simulink model "FootVelocityCalculator"  (R2016b)
settings: Solver=VariableStepAuto  StartTime=0.0  StopTime=10.0  RelTol=1e-3
settings Model: DataDictionary=DataDictionary.sldd  Creator=Taeke  LastModifiedBy=Nathan

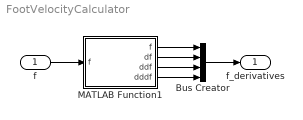
== system FootVelocityCalculator ==
  f : Inport  PortDimensions=numberSamplePoints
  Bus Creator : BusCreator  Inputs='f','df','ddf','dddf'  OutDataTypeStr=Bus: hip
  MATLAB Function1 : MATLAB Function  TreatAsAtomicUnit=on
  f_derivatives : Outport  OutDataTypeStr=Bus: hip
  wires:
  MATLAB Function1/1(f) -> Bus Creator/1
  MATLAB Function1/3(ddf) -> Bus Creator/3
  MATLAB Function1/2(df) -> Bus Creator/2
  MATLAB Function1/4(dddf) -> Bus Creator/4
  f/1 -> MATLAB Function1/1("f ")
  Bus Creator/1 -> f_derivatives/1

== matlab function FootVelocityCalculator/MATLAB Function1 ==
  data: f input; f output; df output; ddf output; dddf output

function [f, df, ddf, dddf] = fcn(f)
t = 0.1*4/100; %[s]
[df, ddf, dddf] = derivatives(f,t);
end
